simulink model "problem5"  (R2020b)
settings: Solver=VariableStepAuto  StartTime=0.0  StopTime=10.0  RelTol=1e-3
model workspace (MAT data in the model file):
  C = Simulink.Parameter
  C.Value = 0.5
  C.DataType = 'auto'
  C.Dimensions = [1 1]
  R = Simulink.Parameter
  R.Value = 120
  R.DataType = 'auto'
  R.Dimensions = [1 1]
settings Model: Creator=k.Raviteja  LastModifiedBy=k.Raviteja

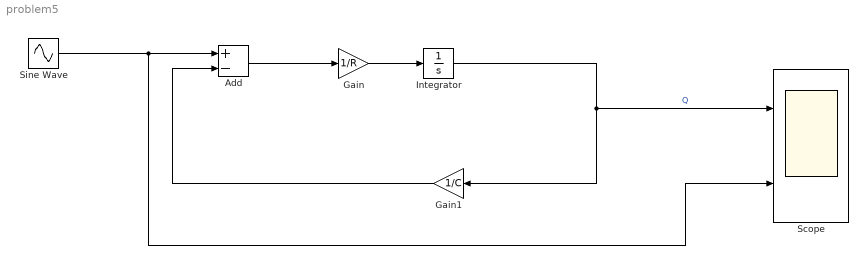
== system problem5 ==
  Add : Sum  Inputs=+-
  Gain : Gain  Gain=1/R
  Gain1 : Gain  Gain=1/C
  Integrator : Integrator
  Scope : Scope  NumInputPorts=2
  Sine Wave : Sin  Samples=1  SampleTime=0
  wires:
  Integrator/1 -> Gain1/1, Scope/1  "Q"
  Gain/1 -> Integrator/1
  Add/1 -> Gain/1
  Gain1/1 -> Add/2
  Sine Wave/1 -> Scope/2, Add/1
